simulink model "Validation"  (R2025a)
settings: Solver=FixedStepAuto  StartTime=0.0  StopTime=10  FixedStep=0.0005  MaxStep=0.01  RelTol=1e-3
values from neighbouring files (symbols this model uses):
  Initial_point = 0    [Matlap_Tuning&Validation.m]    (also in Matlap_Tuning_Validation.m = test_initials(test_idx); tuning_validation_game.m)
  kd_value = 0    [Matlap_Tuning&Validation.m]    (also in Matlap_Tuning_Validation.m = 1.8856)
  ki_value = 0    [Matlap_Tuning&Validation.m]    (also in Matlap_Tuning_Validation.m = 1.3254)
  kp_value = kp_vector(i)    [Matlap_Tuning&Validation.m]    (also in Matlap_Tuning_Validation.m = 3.6237)
  Setpoint = 90    [Matlap_Tuning&Validation.m]    (also in Matlap_Tuning_Validation.m = test_setpoints(test_idx); tuning_validation_game.m = 180)
undefined symbols (not defined in the file or in its folder): Controller_Method, feed_forward, g, J, ke, kt, L, Lm, mp, R, T, X, Y, Z
libraries: sm_lib x14, nesl_utility x4, slpidlib x2
(part 1 of 2)
settings Model: Creator=User  LastModifiedBy=ACER
settings RTWCC: GPUComputeCapability=3.5

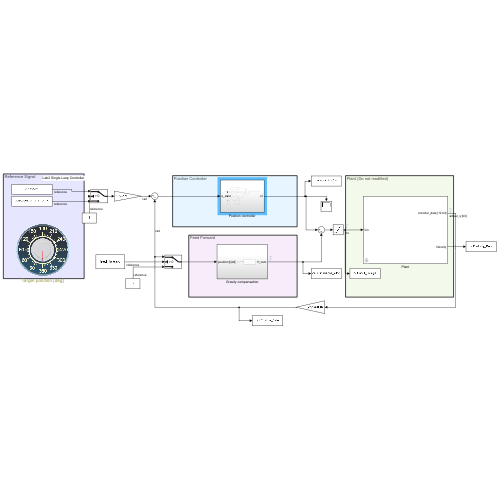
[thumbnail: Simulink's stored preview of the top-level diagram]
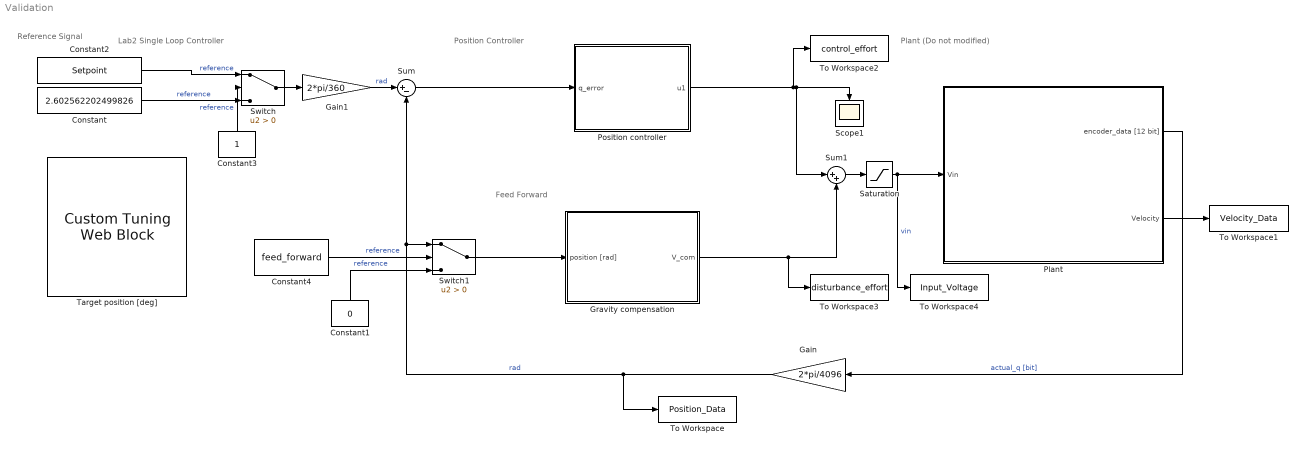
== system Validation ==
  note: Lab2 Single Loop Controller
  note: Plant (Do not modified)
  note: Feed Forward
  note: Position Controller
  note: Reference Signal
  Constant : Constant  Value=2.602562202499826  SampleTime=-1
  Constant1 : Constant  Value=0  SampleTime=-1
  Constant2 : Constant  Value=Setpoint  SampleTime=-1
  Constant3 : Constant  SampleTime=-1
  Constant4 : Constant  Value=feed_forward  SampleTime=-1
  Gain : Gain  Gain=2*pi/4096
  Gain1 : Gain  Gain=2*pi/360
  Gravity compensation : Subsystem
  Plant : Subsystem  mask{init_q=Initial_point}
      mask prompts: init_q "Initial angle of pendulum [deg]"
  Position controller : Subsystem
  Saturation : Saturate  UpperLimit=12  LowerLimit=-12
  Scope1 : Scope
      settings: ActiveDisplayYMinimum=-4.6716407537940983  ActiveDisplayYMaximum=3.7178741740051438
  Sum : Sum  Inputs=|+-
  Sum1 : Sum  Inputs=|++
  Switch : Switch  Criteria=u2 > Threshold  SaturateOnIntegerOverflow=off  InputSameDT=off
  Switch1 : Switch  Criteria=u2 > Threshold  SaturateOnIntegerOverflow=off  InputSameDT=off
  Target position [deg] : CustomTuningWebBlock  LabelPosition=Hide  ShowInitialText=on  Configuration="{\"components\":[{\"name\":\"CircularScaleComponent\",\"settings\":{\"bounds\":{\"max\":360,\"min\":0,\"tickInterval\":30},\"direction\":\"cw\",\"flipLimits\":0,\"innerRadius\":0.6636618227670849,\"internalTickHeightScaleFactor\":1,\"labelColor\":[255,255,200],\"labelFont\":{\"font\":\"Arial\",\"fontSize\":12},\"labelRadius\":0.79,\"labelTransparency\":1,\"minorTickHeightScaleFactor\":0.2,\"needleImage\":{\"size\":[150,150],\"src\":\"data:image\\/svg+xml;base64,PD94bWwgdmVyc2lvbj0iMS4wIiBlbmNvZGluZz0idXRmLTgiPz4NCjwhLS0gR2VuZXJhdG9yOiBBZG9iZSBJbGx1c3RyYXRvciAyNS4yLjMsIFNWRyBFeHBvcnQgUGx1Zy1JbiAuIFNWRyBWZXJzaW9uOiA2LjAwIEJ1aWxkIDApICAtLT4NCjxzdmcgdmVyc2lvbj0iMS4xIiBpZD0iTGF5ZXJfMSIgeG1sbnM9Imh0dHA6Ly93d3cudzMub3JnLzIwMDAvc3ZnIiB4bWxuczp4bGluaz0iaHR0cDovL3d3dy53My5vcmcvMTk5OS94bGluayIgeD0iMHB4IiB5PSIwcHgiDQoJIHZpZXdCb3g9IjAgMCAxNTIgMTUyIiBzdHlsZT0iZW5hYmxl ...(+37472 chars)\"},\"needleOffset\":[0,0],\"needleOrientation\":-45,\"needleRotation\":90,\"needleSize\":{\"height\":0.44,\"width\":0.44},\"outerRadius\":0.5053386200069245,\"position\":[0,0,1,1],\"referencePoint\":\"auto\",\"scaleAngle\":360,\"scaleAngleOffset\":90,\"scaleColors\":[],\"scaleColorsSize\":0.2,\"scaleDirection\":\"CW\",\"scalePosition\":[0,0,1,1],\"showLabels\":1,\"showMinorTicks\":1,\"showSpanLine\":true,\"showTicks\":1,\"tickColor\":[252,252,197],\"tickTransparency\":1,\"valueBarColor\":[0,114,189],\"valueBarPosition\":[0,0,1,1],\"valueBarSize\":0.2,\"valueBarTransparency\":1}},{\"name\":\"BackgroundImageComponent\",\"settings\":{\"image\":{\"size\":[385,373],\"src\":\"data:image\\/svg+xml;base64,PD94bWwgdmVyc2lvbj0iMS4wIiBlbmNvZGluZz0idXRmLTgiPz4NCjwhLS0gR2VuZXJhdG9yOiBBZG9iZSBJbGx1c3RyYXRvciAyNS4wLjAsIFNWRyBFeHBvcnQgUGx1Zy1JbiAuIFNWRyBWZXJzaW9uOiA2LjAwIEJ1aWxkIDApICAtLT4NCjxzdmcgdmVyc2lvbj0iMS4xIg0KCSBpZD0iTGF5ZXJfMl8xXyIgeG1sbnM6Y2M9Imh0dHA6Ly9jcmVhdGl2ZWNvbW1vbnMub3JnL25zIyIgeG1sbnM6ZGM9Imh0dHA6Ly9wdXJsLm9yZy9kYy9lbGVtZW50cy8xLjEvIiB4bWxuczppbmtzY2FwZT0iaHR0cDovL3d3dy5pbmtzY2FwZS5vcmcv ...(+4184 chars)\",\"srcOrientation\":\"horizontal\"},\"position\":[0,0,1,1],\"scaleMode\":\"0\"}},{\"name\":\"ForegroundImageComponent\",\"settings\":{\"image\":{\"size\":[0,0],\"src\":\"default\",\"srcOrientation\":[]},\"isForeground\":1,\"position\":[0,0,1,1],\"scaleMode\":\"0\"}}],\"derived\":{\"blockParameters\":{\"ForegroundColor\":[0.9882352941176471,0.9882352941176471,0.7725490196078432],\"Limits\":{\"Max\":360,\"Min\":0,\"Ticks\":30},\"ScaleColors\":[],\"ScaleDirection\":\"Clockwise\",\"ScaleMax\":360,\"ScaleMin\":0,\"TickInterval\":30,\"fixedAspectRatio\":\"off\"}},\"settings\":{\"BindingType\":\"param\",\"aspectRatio\":1,\"backgroundColor\":[0,0,0,\"1\"],\"backgroundOffset\":1,\"backgroundOpacity\":1,\"direction\":\"cw\",\"fixedAspectRatio\":\"off\",\"flipLimits\":0,\"foregroundColor\":[252,252,196],\"orientation\":\"horizontal\",\"showBackgroundColor\":false,\"value\":0,\"version\":\"R2023a\"},\"type\":\"CircularGauge\"}"
  To Workspace : ToWorkspace  VariableName=Position_Data  SaveFormat=Timeseries  SampleTime=-1
  To Workspace1 : ToWorkspace  VariableName=Velocity_Data  SaveFormat=Timeseries  SampleTime=-1
  To Workspace2 : ToWorkspace  VariableName=control_effort  SaveFormat=Timeseries  SampleTime=-1
  To Workspace3 : ToWorkspace  VariableName=disturbance_effort  SaveFormat=Timeseries  SampleTime=-1
  To Workspace4 : ToWorkspace  VariableName=Input_Voltage  SaveFormat=Timeseries  SampleTime=-1
  wires:
  Saturation/1 -> Plant/1(Vin), To Workspace4/1  "vin"
  Constant/1 -> Switch/3  "reference"
  Position controller/1(u1) -> To Workspace2/1, Sum1/1, Scope1/1
  Plant/1(encoder_data [12 bit]) -> Gain/1  "actual_q [bit]"
  Sum1/1 -> Saturation/1
  Gain/1 -> To Workspace/1, Switch1/1, Sum/2  "rad"
  Gain1/1 -> Sum/1  "rad"
  Switch/1 -> Gain1/1
  Constant2/1 -> Switch/1  "reference"
  Constant3/1 -> Switch/2  "reference"
  Sum/1 -> Position controller/1(q_error)
  Switch1/1 -> Gravity compensation/1(position [rad])
  Constant1/1 -> Switch1/3  "reference"
  Constant4/1 -> Switch1/2  "reference"
  Plant/2(Velocity) -> To Workspace1/1
  Gravity compensation/1(V_com) -> To Workspace3/1, Sum1/2

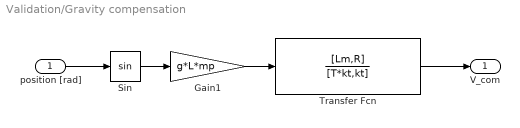
== system Validation/Gravity compensation ==
  position [rad] : Inport
  Gain1 : Gain  Gain=g*L*mp
  Sin : Trigonometry
  Transfer Fcn : TransferFcn  Numerator=[Lm,R]  Denominator=[T*kt,kt]
  V_com : Outport
  wires:
  position [rad]/1 -> Sin/1
  Transfer Fcn/1 -> V_com/1
  Sin/1 -> Gain1/1
  Gain1/1 -> Transfer Fcn/1

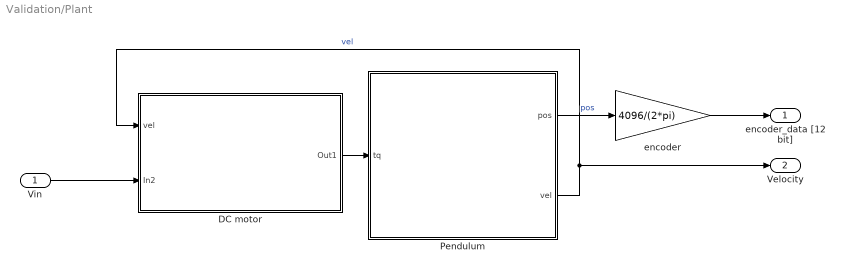
== system Validation/Plant ==
  Vin : Inport
  DC motor : Subsystem
  Pendulum : Subsystem
      mask Display: image('simple_pendulum_brick.png'); % Use "Edit Image" on toolstrip to change.
  encoder : Gain  Gain=4096/(2*pi)
  encoder_data [12 bit] : Outport
  Velocity : Outport  Port=2
  wires:
  Pendulum/1(pos) -> encoder/1  "pos"
  encoder/1 -> encoder_data [12 bit]/1
  Pendulum/2(vel) -> DC motor/1(vel), Velocity/1  "vel"
  Vin/1 -> DC motor/2(In2)
  DC motor/1(Out1) -> Pendulum/1(tq)
